simulink model "KD_cl_harness_tomasso"  (R2014b)
settings: Solver=ode45  StartTime=0  StopTime=50  FixedStep=0.01  MaxStep=0.005  RelTol=1e-4  AbsTol=1e-4
InitFcn:
  | load KD_const_coeffs_0624
  | load pexhat_stuff
  | load expcon
  | load thr_ff_map
values from neighbouring files (symbols this model uses):
  c_0 = 0    [expcon.mat]
  c_1 = 1    [expcon.mat]
  c_100 = 100    [expcon.mat]
  c_1000 = 1000    [expcon.mat]
  c_10000 = 10000    [expcon.mat]
  c_1000inv = 0.0010000000475    [expcon.mat]    (also in pexhat_stuff.mat)
  c_100inv = 0.00999999977648    [expcon.mat]
  c_1_int = 1    [expcon.mat]
  c_1d2p4 = 0.416666656733    [expcon.mat]
  c_1p7 = 1.70000004768    [expcon.mat]
  c_4400inv = 0.000227272728807    [pexhat_stuff.mat]
  c_5500inv = 0.000181818177225    [expcon.mat]
  c_80 = 80    [expcon.mat]
  c_90 = 90    [expcon.mat]
  c_cal_phi = 7.6395999713e-06    [expcon.mat]
  c_compmap = [28125.0058594 29577.4082031 31350.1035156 33776.21875 37051.9296875 41026.2695312 45453.9960938 50160.3515625 55029.671875 59986.109375 64980.4296875 69980.4375 ... (320 elements, 20x16)]    [expcon.mat]
  c_ctok = 273.149993896    [expcon.mat]
  c_fflow_max = inf    [expcon.mat]
  c_fflow_min = 0    [expcon.mat]
  c_filt = 0.949999988079    [expcon.mat]
  c_flowdiv = 9.99999974738e-05    [expcon.mat]
  c_flowmin = 0    [expcon.mat]
  c_flowmult = 10000    [expcon.mat]
  c_inf = inf    [expcon.mat]
  c_km1d2k = 0.142857149243    [expcon.mat]
  c_mm3tokgpers = 2.77333338516e-08    [expcon.mat]
  c_n1 = -1    [expcon.mat]
  c_p00001 = 9.99999974738e-06    [expcon.mat]
  c_p01 = 0.00999999977648    [pexhat_stuff.mat]
  c_p016 = 0.01600000076    [expcon.mat]
  c_p1429 = 0.142900004983    [expcon.mat]
  c_p1e9 = 9.99999971718e-10    [expcon.mat]
  c_p4167 = 0.416700005531    [expcon.mat]    (also in pexhat_stuff.mat = 0.416666656733)
  c_p4d1p4 = 0.285714298487    [expcon.mat]
  c_p5401 = 0.540099978447    [expcon.mat]
  c_p9 = 0.899999976158    [expcon.mat]
  c_pincomp = 97.4216003418    [expcon.mat]
  c_ra = 287.002807617    [expcon.mat]
  c_rair = 287.09979248    [expcon.mat]
  c_Rby1000 = 0.000287000002572    [expcon.mat]
  c_roacorr = 8.05689978733e-06    [expcon.mat]
  c_rpmtoradpers = 0.104719758034    [expcon.mat]
  c_svrthrottle1 = [0.924875080585 0.575991511345 0.0858279466629 0.820202827454 0.445821881294 0.509882986546 0.0428557097912 0.753634572029 0]    [expcon.mat]
  c_svrthrottle2 = [0.145454958081 0.14545533061 0.363636374474 0.509091556072 0.509090721607 0.509091317654 0.545454084873 0.618182241917 0.145454272628]    [expcon.mat]
  c_svrthrottlearg = 0.10000000149    [expcon.mat]
  c_svrthrottlebeta = [2282.12670898 -3239.46044922 -142.784469604 -2660.34570312 1434.34350586 4150.43994141 -1580.68164062 -1039.89575195 791.34588623]    [expcon.mat]
  c_ta_max = inf    [expcon.mat]
  c_ta_min = 270    [expcon.mat]
  c_V = 0.0077999997884    [expcon.mat]
  c_vnliftmax = 90    [expcon.mat]
  c_vnliftmin = 40    [expcon.mat]
  Coefs =     [KD_const_coeffs_0624.mat]    (also in pexhat_stuff.mat)
  const =     [KD_const_coeffs_0624.mat]    (also in pexhat_stuff.mat)
  const_exhat =     [pexhat_stuff.mat]
  eegr_map =     [expcon.mat]
  egrr_delay_init = 0    [expcon.mat]
  epim_map =     [expcon.mat]
  eplufin_ff_map =     [expcon.mat]
  expcon =     [expcon.mat]
  invta = [5 5 5 5 2.5 0 0 0 0 0 0 0 ... (240 elements, 16x15)]    [expcon.mat]
  invtacols = [1000 1200 1400 1600 1800 2000 2200 2400 2600 2800 3000 3200 ... (16 elements, 1x16)]    [expcon.mat]
  IV =     [KD_const_coeffs_0624.mat]    (also in pexhat_stuff.mat)
  Lobs_init = [0 0 0]    [expcon.mat]
  map_delay_init = 120    [expcon.mat]
  maxA_t = [51.4567184448 53.8593139648 56.3063011169 58.7576789856 61.1701469421 63.4982337952 65.6955718994 67.7161483765 69.5156555176 71.0527648926 72.2902603149 73.1961746216 ... (16 elements, 1x16)]    [expcon.mat]
  obsA = [0.985195398331  0  0; -0.188821405172  1  0; 0.000342977960827  0  1]    [expcon.mat]
  sample_time = 0.016    [expcon.mat]    (also in pexhat_stuff.mat)
  SVR_EGR =     [KD_const_coeffs_0624.mat]    (also in pexhat_stuff.mat)
  SVR_EGR_exhat =     [pexhat_stuff.mat]
  SVR_throttle =     [KD_const_coeffs_0624.mat]    (also in pexhat_stuff.mat)
  uz_init = [0 0]    [expcon.mat]
undefined symbols (not defined in the file or in its folder): k1_table, k2_table, maxL, minL, Newton, Raphson
libraries: simulink x5
(part 5 of 6)

== system KD_cl_harness_tomasso/ctrl_rb_explicit_20131031_v2/EGR_max_flow/Air_Model_map_use/Forward_Flow ==
  Ro_a : Inport
  Ne_rpm : Inport  Port=2
  Pa : Inport  Port=3
  Pm : Inport  Port=4
  Cal_phi : Subsystem
  Constant2 : Constant  Value=c_p1429  OutDataTypeStr=single
      settings: AttributesFormatString=%<Value>
  Constant3 : Constant  Value=c_1  OutDataTypeStr=single
      settings: AttributesFormatString=%<Value>
  Constant4 : Constant  Value=c_p5401  OutDataTypeStr=single
      settings: AttributesFormatString=%<Value>
  Constant5 : Constant  Value=c_p4167  OutDataTypeStr=single
      settings: AttributesFormatString=%<Value>
  Lookup Table : Lookup  InputValues=invtacols  Table=maxA_t
  Pm_by_Pa : Product  Inputs=*/  SaturateOnIntegerOverflow=on  RndMeth=Zero  InputSameDT=on  OutDataTypeStr=Inherit: Same as first input
  Relational Operator : RelationalOperator  Operator=>  OutDataTypeStr=boolean
      settings: AttributesFormatString=%<Operator>
  Saturation1 : Saturate  UpperLimit=c_1  LowerLimit=c_p4167
      settings: AttributesFormatString=%<UpperLimit>\n%<LowerLimit>
  Saturation2 : Saturate  UpperLimit=c_inf  LowerLimit=c_0
      settings: AttributesFormatString=%<LowerLimit>\n%<UpperLimit>
  Saturation3 : Saturate  UpperLimit=c_inf  LowerLimit=c_100
      settings: AttributesFormatString=%<LowerLimit>\n%<UpperLimit>
  Sqrt : Sqrt  AlgorithmType=Newton-Raphson  SaturateOnIntegerOverflow=on
  Sum : Sum  Inputs=|+-
  Sum1 : Sum  Inputs=|++
  Switch1 : Switch  Criteria=u2 ~= 0
      settings: AttributesFormatString=%<Criteria>
  correct flow1 : Product  Inputs=**  SaturateOnIntegerOverflow=on  RndMeth=Zero  InputSameDT=on  OutDataTypeStr=Inherit: Same as first input
  correct flow2 : Product  Inputs=***  SaturateOnIntegerOverflow=on  RndMeth=Zero  InputSameDT=on  OutDataTypeStr=Inherit: Same as first input
  correct flow3 : Product  Inputs=**  SaturateOnIntegerOverflow=on  RndMeth=Zero  InputSameDT=on  OutDataTypeStr=Inherit: Same as first input
  tokgps1 : Gain  Gain=c_1000inv
  mt_dot_kg_per_s : Outport
  wires:
  Sqrt/1 -> Switch1/1
  correct flow3/1 -> Saturation2/1
  correct flow1/1 -> Sum1/1
  Constant2/1 -> correct flow1/2
  Sum/1 -> correct flow3/1, correct flow1/1
  Constant3/1 -> Sum/1
  Lookup Table/1 -> correct flow2/2  "B_TA"
  Ne_rpm/1 -> Lookup Table/1
  Ro_a/1 -> Cal_phi/2(Ro_a)
  Pa/1 -> [Pa], Saturation3/1
  Pm/1 -> Pm_by_Pa/1
  Pm_by_Pa/1 -> Saturation1/1, Relational Operator/1
  tokgps1/1 -> mt_dot_kg_per_s/1
  correct flow2/1 -> tokgps1/1
  Saturation1/1 -> Sum1/2, Sum/2
  Switch1/1 -> correct flow2/3
  Cal_phi/1(phi) -> correct flow2/1
  Sum1/1 -> correct flow3/2
  [Pa] -> Cal_phi/1(Pa)
  Saturation2/1 -> Sqrt/1
  Saturation3/1 -> Pm_by_Pa/2
  Relational Operator/1 -> Switch1/2
  Constant4/1 -> Switch1/3
  Constant5/1 -> Relational Operator/2

== system KD_cl_harness_tomasso/ctrl_rb_explicit_20131031_v2/While_Iterator_Subsystem/newton/For_Iterator_Subsystem ==
  u : Inport
  sv1 : Inport  Port=2
  sv2 : Inport  Port=3
  arg : Inport  Port=4
  beta : Inport  Port=5
  Demux : Demux  Outputs=2
  Divide : Product  Inputs=*/
  For Iterator : ForIterator  ResetStates=reset  IterationLimit=SVR_EGR_exhat.num_SV
  Gain : Gain  Gain=100
      settings: AttributesFormatString=%<Gain>
  Product{,1..3} (4 alike) : Product  RndMeth=Zero
  Saturation1 : Saturate  UpperLimit=9  LowerLimit=1
      settings: AttributesFormatString=%<LowerLimit>\n%<UpperLimit>
  Selector : Selector  InputPortWidth=SVR_EGR_exhat.num_SV  IndexOptions=Index vector (port)  Indices=[1 3]
  Selector1 : Selector  InputPortWidth=SVR_EGR_exhat.num_SV  IndexOptions=Index vector (port)  Indices=[1 3]
  Selector2 : Selector  InputPortWidth=SVR_EGR_exhat.num_SV  IndexOptions=Index vector (port)  Indices=[1 3]
  Sum : Sum  Inputs=|-+
  Sum1 : Sum  Inputs=+-|
  Sum2 : Sum  Inputs=-|-
  Sum3 : Sum  Inputs=++|
  Unit Delay : UnitDelay  SampleTime=-1
  exp Lookup Table : Lookup  InputValues=SVR_EGR_exhat.exp.x  Table=SVR_EGR_exhat.exp.y  LookUpMeth=Interpolation-Use End Values
      settings: AttributesFormatString=%<LookUpMeth>\n%<InputValues>
  ba : Outport  OutDataTypeStr=single
  wires:
  Saturation1/1 -> [iter]
  For Iterator/1 -> Saturation1/1
  [iter] -> Selector2/2
  [iter] -> Selector1/2
  [iter] -> Selector/2
  Sum3/1 -> ba/1, Unit Delay/1
  Product3/1 -> Sum3/2
  Selector2/1 -> Product3/2
  Gain/1 -> Divide/2
  Product2/1 -> Gain/1
  arg/1 -> Product2/2, Product2/1
  Sum2/1 -> Divide/1
  Product1/1 -> Sum2/2
  Product/1 -> Sum2/1
  Sum1/1 -> Product1/2, Product1/1
  Sum/1 -> Product/2, Product/1
  Demux/2 -> Sum1/1
  Selector1/1 -> Sum1/2
  Demux/1 -> Sum/2
  Selector/1 -> Sum/1
  u/1 -> Demux/1
  beta/1 -> Selector2/1
  sv2/1 -> Selector1/1
  sv1/1 -> Selector/1
  Unit Delay/1 -> Sum3/1
  Divide/1 -> exp Lookup Table/1
  exp Lookup Table/1 -> Product3/1

== system KD_cl_harness_tomasso/ctrl_rb_explicit_20131031_v2/While_Iterator_Subsystem/newton/If_Action_Subsystem ==
  pex : Inport
  ba : Inport  Port=2
  c : Inport  Port=3
  k : Inport  Port=4
  Action Port : ActionPort  ActionType=then
  Gain1 : Gain  Gain=2
  Gain6 : Gain  Gain=2
  Mux : Mux  Inputs=2
  Product : Product  Inputs=***  RndMeth=Zero
  Product1 : Product  Inputs=*/  RndMeth=Zero
  Product2 : Product  Inputs=**  RndMeth=Zero
  Product3 : Product  Inputs=***  RndMeth=Zero
  Product4 : Product  Inputs=*/  RndMeth=Zero
  Saturation1 : Saturate  UpperLimit=inf  LowerLimit=0
      settings: AttributesFormatString=%<LowerLimit>\n%<UpperLimit>
  Saturation2 : Saturate  UpperLimit=inf  LowerLimit=0
      settings: AttributesFormatString=%<LowerLimit>\n%<UpperLimit>
  Saturation3 : Saturate  UpperLimit=c_inf  LowerLimit=c_p1e9
      settings: AttributesFormatString=%<LowerLimit>\n%<UpperLimit>
  Saturation4 : Saturate  UpperLimit=c_inf  LowerLimit=c_p1e9
      settings: AttributesFormatString=%<LowerLimit>\n%<UpperLimit>
  Sqrt1 : Sqrt  AlgorithmType=Newton-Raphson  SaturateOnIntegerOverflow=on
  Sqrt2 : Sqrt  AlgorithmType=Newton-Raphson  SaturateOnIntegerOverflow=on
  Sum1 : Sum  Inputs=++|
  Sum3 : Sum  Inputs=++|
  one : Constant  OutDataTypeStr=single  SampleTime=-1
      settings: AttributesFormatString=%<Value>\n%<SampleTime>
  one1 : Constant  OutDataTypeStr=single  SampleTime=-1
      settings: AttributesFormatString=%<Value>\n%<SampleTime>
  Out : Outport
  wires:
  Saturation4/1 -> Product4/2
  Saturation3/1 -> Product1/2
  Saturation2/1 -> Sqrt1/1
  Saturation1/1 -> Sqrt2/1
  Product3/1 -> Product2/1
  Sqrt1/1 -> Product3/3
  Product4/1 -> Saturation2/1
  Gain1/1 -> Saturation4/1
  Sum1/1 -> Gain1/1
  one1/1 -> Sum1/1
  [k] -> Sum1/2
  [k] -> Product4/1
  [c] -> Product3/2
  [ba] -> Product3/1
  Mux/1 -> Out/1
  Product2/1 -> Mux/2
  Product/1 -> Mux/1
  Sqrt2/1 -> Product/3
  [pex] -> Product2/2
  Product1/1 -> Saturation1/1
  Gain6/1 -> Saturation3/1
  Sum3/1 -> Gain6/1
  one/1 -> Sum3/1
  [k] -> Sum3/2
  [k] -> Product1/1
  [c] -> Product/2
  [ba] -> Product/1
  k/1 -> [k]
  pex/1 -> [pex]
  c/1 -> [c]
  ba/1 -> [ba]

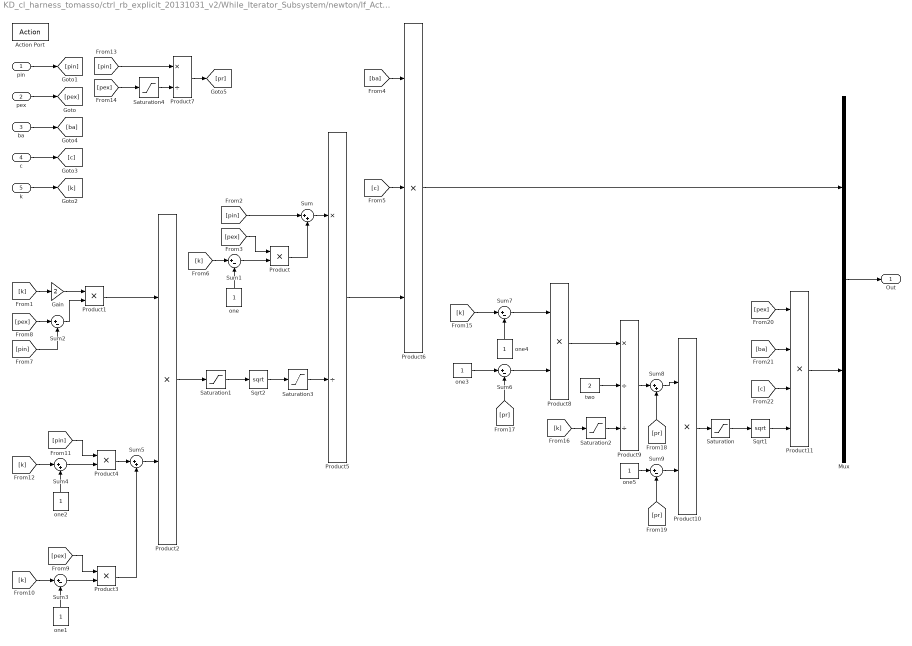
== system KD_cl_harness_tomasso/ctrl_rb_explicit_20131031_v2/While_Iterator_Subsystem/newton/If_Action_Subsystem1 ==
  pin : Inport
  pex : Inport  Port=2
  ba : Inport  Port=3
  c : Inport  Port=4
  k : Inport  Port=5
  Action Port : ActionPort  ActionType=else
  Gain : Gain  Gain=2
  Mux : Mux  Inputs=2
  Product{,1..4} (5 alike) : Product  RndMeth=Zero
  Product10 : Product  Inputs=**  RndMeth=Zero
  Product11 : Product  Inputs=****  RndMeth=Zero
  Product5 : Product  Inputs=*/  RndMeth=Zero
  Product6 : Product  Inputs=***  RndMeth=Zero
  Product7 : Product  Inputs=*/  RndMeth=Zero
  Product8 : Product  Inputs=**  RndMeth=Zero
  Product9 : Product  Inputs=*//  RndMeth=Zero
  Saturation : Saturate  UpperLimit=inf  LowerLimit=0
      settings: AttributesFormatString=%<LowerLimit>\n%<UpperLimit>
  Saturation1 : Saturate  UpperLimit=inf  LowerLimit=0
      settings: AttributesFormatString=%<LowerLimit>\n%<UpperLimit>
  Saturation2 : Saturate  UpperLimit=c_inf  LowerLimit=c_p1e9
      settings: AttributesFormatString=%<LowerLimit>\n%<UpperLimit>
  Saturation3 : Saturate  UpperLimit=c_inf  LowerLimit=c_p00001
      settings: AttributesFormatString=%<LowerLimit>\n%<UpperLimit>
  Saturation4 : Saturate  UpperLimit=c_inf  LowerLimit=c_p1e9
      settings: AttributesFormatString=%<LowerLimit>\n%<UpperLimit>
  Sqrt1 : Sqrt  AlgorithmType=Newton-Raphson  SaturateOnIntegerOverflow=on
  Sqrt2 : Sqrt  AlgorithmType=Newton-Raphson  SaturateOnIntegerOverflow=on
  Sum{,4..5,8} (4 alike) : Sum  Inputs=|++
  Sum{1..3,6..7,9} (6 alike) : Sum  Inputs=|+-
  one{,1..5} (6 alike) : Constant  OutDataTypeStr=single  SampleTime=-1
      settings: AttributesFormatString=%<Value>\n%<SampleTime>
  two : Constant  Value=2  OutDataTypeStr=single  SampleTime=-1
      settings: AttributesFormatString=%<Value>\n%<SampleTime>
  Out : Outport
  wires:
  Saturation4/1 -> Product7/2
  Saturation2/1 -> Product9/3
  Saturation1/1 -> Sqrt2/1
  Saturation/1 -> Sqrt1/1
  Mux/1 -> Out/1
  Product6/1 -> Mux/1
  Product11/1 -> Mux/2
  [c] -> Product11/3
  [ba] -> Product11/2
  [pex] -> Product11/1
  Sqrt1/1 -> Product11/4
  Product10/1 -> Saturation/1
  Sum8/1 -> Product10/1
  [pr] -> Sum9/2
  Sum9/1 -> Product10/2
  one5/1 -> Sum9/1
  [pr] -> Sum8/2
  Product9/1 -> Sum8/1
  [pr] -> Sum6/2
  Product7/1 -> [pr]
  [k] -> Saturation2/1
  two/1 -> Product9/2
  Product8/1 -> Product9/1
  Sum7/1 -> Product8/1
  Sum6/1 -> Product8/2
  one4/1 -> Sum7/2
  [k] -> Sum7/1
  [pex] -> Saturation4/1
  [pin] -> Product7/1
  one3/1 -> Sum6/1
  Product5/1 -> Product6/3
  [c] -> Product6/2
  [ba] -> Product6/1
  Sum/1 -> Product5/1
  Sqrt2/1 -> Saturation3/1
  Product2/1 -> Saturation1/1
  Product3/1 -> Sum5/2
  Product4/1 -> Sum5/1
  Sum5/1 -> Product2/2
  [pin] -> Product4/1
  Sum4/1 -> Product4/2
  [k] -> Sum4/1
  one2/1 -> Sum4/2
  [pex] -> Product3/1
  Sum3/1 -> Product3/2
  [k] -> Sum3/1
  one1/1 -> Sum3/2
  Product1/1 -> Product2/1
  Gain/1 -> Product1/1
  Sum2/1 -> Product1/2
  [pex] -> Sum2/1
  [pin] -> Sum2/2
  [k] -> Gain/1
  Product/1 -> Sum/2
  [pex] -> Product/1
  Sum1/1 -> Product/2
  [k] -> Sum1/1
  one/1 -> Sum1/2
  [pin] -> Sum/1
  pin/1 -> [pin]
  k/1 -> [k]
  c/1 -> [c]
  ba/1 -> [ba]
  pex/1 -> [pex]
  Saturation3/1 -> Product5/2

== system KD_cl_harness_tomasso/ctrl_rb_explicit_20131031_v2/While_Iterator_Subsystem/newton/If_Action_Subsystem2 ==
  pex_hat : Inport
  Action Port : ActionPort  ActionType=else
  pex : Outport
  wires:
  pex_hat/1 -> pex/1

== system KD_cl_harness_tomasso/ctrl_rb_explicit_20131031_v2/While_Iterator_Subsystem/newton/If_Action_Subsystem3 ==
  valve : Inport
  pex_hat : Inport  Port=2
  pex_ecu : Inport  Port=3
  Action Port : ActionPort  ActionType=then
  Divide : Product  Inputs=*/
  Divide1 : Product  Inputs=**
  Divide2 : Product  Inputs=**
  Sum : Sum  Inputs=-+|
  Sum1 : Sum  Inputs=+|+
  fifteen : Constant  Value=15  OutDataTypeStr=single
      settings: AttributesFormatString=%<Value>
  one : Constant  OutDataTypeStr=single
      settings: AttributesFormatString=%<Value>
  pex : Outport
  wires:
  valve/1 -> Divide/1
  fifteen/1 -> Divide/2
  Divide/1 -> Divide1/2, Sum/1
  pex_hat/1 -> Divide1/1
  one/1 -> Sum/2
  Sum/1 -> Divide2/1
  pex_ecu/1 -> Divide2/2
  Divide1/1 -> Sum1/1
  Divide2/1 -> Sum1/2
  Sum1/1 -> pex/1

== system KD_cl_harness_tomasso/ctrl_rb_explicit_20131031_v2/While_Iterator_Subsystem/newton/update ==
  dwdp : Inport
  error : Inport  Port=2
  Data Store Read1 : DataStoreRead  DataStoreName=man_pex_eps
  Data Store Read11 : DataStoreRead  DataStoreName=man_pex_eps
  Data Store Read16 : DataStoreRead  DataStoreName=man_use_LM
  Product2 : Product  Inputs=**  RndMeth=Zero
  Product3 : Product  Inputs=/*  RndMeth=Zero
  Product8 : Product  Inputs=/**  RndMeth=Zero
  Relational Operator7 : RelationalOperator  Operator=>  OutDataTypeStr=boolean
      settings: AttributesFormatString=%<Operator>
  Saturation1 : Saturate  UpperLimit=c_inf  LowerLimit=c_p1e9
      settings: AttributesFormatString=%<LowerLimit>\n%<UpperLimit>
  Saturation3 : Saturate  UpperLimit=c_inf  LowerLimit=c_p1e9
      settings: AttributesFormatString=%<LowerLimit>\n%<UpperLimit>
  Sum1 : Sum  Inputs=|++
  Sum2 : Sum  Inputs=|++
  Switch7 : Switch  Criteria=u2 ~= 0
      settings: AttributesFormatString=%<Criteria>
  man_pex_eps : Gain
  man_pex_eps1 : Gain
  man_use_LM : Gain
  zero8 : Constant  Value=0  OutDataTypeStr=single  SampleTime=-1
      settings: AttributesFormatString=%<Value>\n%<SampleTime>
  delta : Outport
  wires:
  Data Store Read11/1 -> man_pex_eps/1
  Sum2/1 -> Saturation3/1
  Saturation3/1 -> Product8/1
  Product2/1 -> Sum2/2
  error/1 -> [e]
  dwdp/1 -> [dwdp]
  [dwdp] -> Product2/1, Product8/2, Product2/2
  [e] -> Product8/3
  Data Store Read1/1 -> man_pex_eps1/1
  Sum1/1 -> Saturation1/1
  Saturation1/1 -> Product3/1
  [dwdp] -> Sum1/2
  [e] -> Product3/2
  zero8/1 -> Relational Operator7/2
  Data Store Read16/1 -> man_use_LM/1
  Relational Operator7/1 -> Switch7/2
  Product3/1 -> Switch7/3
  Product8/1 -> Switch7/1
  Switch7/1 -> delta/1
  man_pex_eps/1 -> Sum2/1
  man_pex_eps1/1 -> Sum1/1
  man_use_LM/1 -> Relational Operator7/1

== system KD_cl_harness_tomasso/ctrl_rb_explicit_20131031_v2/expcon/find_region/find_region ==
  u : Inport
  IC : Inport  Port=2
  Constant : Constant  DisableCoverage=on  Value=c_0  OutDataTypeStr=Inherit: Inherit via back propagation  PreserveConstantTs=on
      settings: AttributesFormatString=%<Value>
  g_zero_continue : RelationalOperator  Operator=>  OutDataTypeStr=boolean  InputSameDT=on
  get_region_violation : Subsystem
  if_region_1 : SwitchCase
  leq_check : Subsystem
  reg_register : UnitDelay  InitialCondition=c_1_int  SampleTime=-1
      settings: AttributesFormatString=%<X0>
  reg_update_merge : Merge  Inputs=3  InitialOutput=c_1_int
      settings: AttributesFormatString=%<InitialOutput>
  region_1feedthrough : Subsystem  TreatAsAtomicUnit=on
  region_iter : WhileIterator  MaxIters=expcon.Nr  ShowIterationPort=on
  rv_register : UnitDelay  InitialCondition=c_10000  SampleTime=-1
      settings: AttributesFormatString=%<X0>
  rv_update_merge : Merge  Inputs=3  InitialOutput=c_10000
      settings: AttributesFormatString=%<InitialOutput>
  region : Outport  InitialOutput=c_1_int
      settings: AttributesFormatString=%<InitialOutput>
  rv : Outport  Port=2  InitialOutput=c_10000
      settings: AttributesFormatString=%<InitialOutput>
  wires:
  region_iter/1 -> [iter]
  [iter] -> if_region_1/1, get_region_violation/1(region), leq_check/2(region_ind)
  IC/1 -> region_iter/2
  Constant/1 -> g_zero_continue/2
  [reg] -> reg_update_merge/1
  region_1feedthrough/2(region) -> [reg]
  [def] -> leq_check/Action
  if_region_1/2 -> [def]
  [u] -> get_region_violation/2(u)
  u/1 -> [u]
  get_region_violation/1(region_violation) -> region_1feedthrough/1(rvin), leq_check/1(rv_new)
  leq_check/1(rv_update_new) -> rv_update_merge/2
  rv_register/1 -> leq_check/3(rv_old)
  g_zero_continue/1 -> region_iter/1
  leq_check/3(region_update_new) -> reg_update_merge/2
  reg_register/1 -> leq_check/4(region_old)
  reg_update_merge/1 -> reg_register/1, region/1
  rv_update_merge/1 -> g_zero_continue/1, rv_register/1, rv/1
  region_1feedthrough/1(rvout) -> rv_update_merge/1
  if_region_1/1 -> region_1feedthrough/Action
  leq_check/2(rv_update_old) -> rv_update_merge/3
  leq_check/4(region_updateold) -> reg_update_merge/3

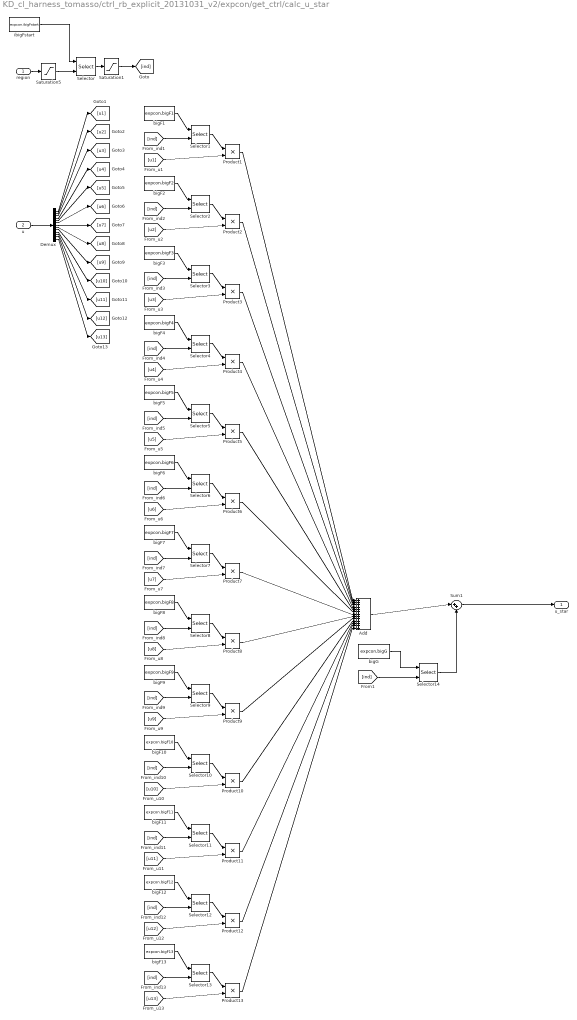
== system KD_cl_harness_tomasso/ctrl_rb_explicit_20131031_v2/expcon/get_ctrl/calc_u_star ==
  region : Inport
  u : Inport  Port=2
  Add : Sum  Inputs=+++++++++++++
  Demux : Demux  Outputs=13
  Product{1..13} (13 alike) : Product  RndMeth=Zero
  Saturation1 : Saturate  UpperLimit=307  LowerLimit=1
      settings: AttributesFormatString=%<LowerLimit>\n%<UpperLimit>
  Saturation5 : Saturate  UpperLimit=103  LowerLimit=1
      settings: AttributesFormatString=%<LowerLimit>\n%<UpperLimit>
  Selector : Selector  InputPortWidth=expcon.Nr  IndexOptions=Index vector (port)  Indices=[1 3]
  Selector{1..14} (14 alike) : Selector  InputPortWidth=309  IndexOptions=Starting index (port)  Indices=[1 3]  OutputSizes=3
  Sum1 : Sum  Inputs=|++
  bigF1 : Constant  Value=expcon.bigF1  OutDataTypeStr=single
      settings: AttributesFormatString=%<Value>
  bigF10 : Constant  Value=expcon.bigF10  OutDataTypeStr=single
      settings: AttributesFormatString=%<Value>
  bigF11 : Constant  Value=expcon.bigF11  OutDataTypeStr=single
      settings: AttributesFormatString=%<Value>
  bigF12 : Constant  Value=expcon.bigF12  OutDataTypeStr=single
      settings: AttributesFormatString=%<Value>
  bigF13 : Constant  Value=expcon.bigF13  OutDataTypeStr=single
      settings: AttributesFormatString=%<Value>
  bigF2 : Constant  Value=expcon.bigF2  OutDataTypeStr=single
      settings: AttributesFormatString=%<Value>
  bigF3 : Constant  Value=expcon.bigF3  OutDataTypeStr=single
      settings: AttributesFormatString=%<Value>
  bigF4 : Constant  Value=expcon.bigF4  OutDataTypeStr=single
      settings: AttributesFormatString=%<Value>
  bigF5 : Constant  Value=expcon.bigF5  OutDataTypeStr=single
      settings: AttributesFormatString=%<Value>
  bigF6 : Constant  Value=expcon.bigF6  OutDataTypeStr=single
      settings: AttributesFormatString=%<Value>
  bigF7 : Constant  Value=expcon.bigF7  OutDataTypeStr=single
      settings: AttributesFormatString=%<Value>
  bigF8 : Constant  Value=expcon.bigF8  OutDataTypeStr=single
      settings: AttributesFormatString=%<Value>
  bigF9 : Constant  Value=expcon.bigF9  OutDataTypeStr=single
      settings: AttributesFormatString=%<Value>
  bigG : Constant  Value=expcon.bigG  OutDataTypeStr=single
      settings: AttributesFormatString=%<Value>
  ibigFstart : Constant  Value=expcon.ibigFstart  OutDataTypeStr=single
      settings: AttributesFormatString=%<Value>
  u_star : Outport
  wires:
  Product13/1 -> Add/13
  [u13] -> Product13/2
  Selector13/1 -> Product13/1
  [ind] -> Selector13/2
  bigF13/1 -> Selector13/1
  Demux/13 -> [u13]
  Product12/1 -> Add/12
  [u12] -> Product12/2
  Selector12/1 -> Product12/1
  [ind] -> Selector12/2
  bigF12/1 -> Selector12/1
  Demux/12 -> [u12]
  Product11/1 -> Add/11
  [u11] -> Product11/2
  Selector11/1 -> Product11/1
  [ind] -> Selector11/2
  bigF11/1 -> Selector11/1
  Demux/11 -> [u11]
  Product10/1 -> Add/10
  [u10] -> Product10/2
  Selector10/1 -> Product10/1
  [ind] -> Selector10/2
  bigF10/1 -> Selector10/1
  Demux/10 -> [u10]
  Product9/1 -> Add/9
  [u9] -> Product9/2
  Selector9/1 -> Product9/1
  [ind] -> Selector9/2
  bigF9/1 -> Selector9/1
  Demux/9 -> [u9]
  Product8/1 -> Add/8
  [u8] -> Product8/2
  Selector8/1 -> Product8/1
  [ind] -> Selector8/2
  bigF8/1 -> Selector8/1
  Demux/8 -> [u8]
  Product7/1 -> Add/7
  [u7] -> Product7/2
  Selector7/1 -> Product7/1
  [ind] -> Selector7/2
  bigF7/1 -> Selector7/1
  Demux/7 -> [u7]
  Product6/1 -> Add/6
  [u6] -> Product6/2
  Selector6/1 -> Product6/1
  [ind] -> Selector6/2
  bigF6/1 -> Selector6/1
  Demux/6 -> [u6]
  Product5/1 -> Add/5
  [u5] -> Product5/2
  Selector5/1 -> Product5/1
  [ind] -> Selector5/2
  bigF5/1 -> Selector5/1
  Demux/5 -> [u5]
  Product4/1 -> Add/4
  [u4] -> Product4/2
  Selector4/1 -> Product4/1
  [ind] -> Selector4/2
  bigF4/1 -> Selector4/1
  Demux/4 -> [u4]
  Product3/1 -> Add/3
  [u3] -> Product3/2
  Selector3/1 -> Product3/1
  [ind] -> Selector3/2
  bigF3/1 -> Selector3/1
  Demux/3 -> [u3]
  Product2/1 -> Add/2
  [u2] -> Product2/2
  Selector2/1 -> Product2/1
  [ind] -> Selector2/2
  bigF2/1 -> Selector2/1
  Demux/2 -> [u2]
  Product1/1 -> Add/1
  [u1] -> Product1/2
  Selector1/1 -> Product1/1
  [ind] -> Selector1/2
  bigF1/1 -> Selector1/1
  Demux/1 -> [u1]
  Saturation1/1 -> [ind]
  Saturation5/1 -> Selector/2
  Add/1 -> Sum1/1
  [ind] -> Selector14/2
  u/1 -> Demux/1
  Selector14/1 -> Sum1/2
  bigG/1 -> Selector14/1
  Sum1/1 -> u_star/1
  Selector/1 -> Saturation1/1
  ibigFstart/1 -> Selector/1
  region/1 -> Saturation5/1

== system KD_cl_harness_tomasso/ctrl_rb_explicit_20131031_v2/invert_flow/valve_inversion/Cal_phi1 ==
  Pa : Inport
  Ro_a : Inport  Port=2
  Abs : Abs
  Gain1 : Gain  Gain=c_cal_phi  SaturateOnIntegerOverflow=on  OutDataTypeStr=Inherit: Same as input  ParamDataTypeStr=Inherit: Same as input
  Product4 : Product  Inputs=**  SaturateOnIntegerOverflow=on  RndMeth=Zero  InputSameDT=on  OutDataTypeStr=Inherit: Same as first input
  Sqrt : Sqrt  AlgorithmType=Newton-Raphson  SaturateOnIntegerOverflow=on
  phi : Outport
  wires:
  Abs/1 -> Sqrt/1
  Gain1/1 -> Abs/1
  Sqrt/1 -> phi/1
  Ro_a/1 -> Product4/2
  Pa/1 -> Product4/1
  Product4/1 -> Gain1/1

== system KD_cl_harness_tomasso/ctrl_rb_explicit_20131031_v2/ntestimator/Throttle_Model/Air_Model_map_use ==
  TA_deg : Inport
  Ne_rpm : Inport  Port=2
  Pim_Pa : Inport  Port=3
  Ta_K : Inport  Port=4
  R_a : Inport  Port=5
  wegrthr : Inport  Port=6
  Forward_Flow : Subsystem
  Product1 : Product  Inputs=*//  SaturateOnIntegerOverflow=on  RndMeth=Zero  InputSameDT=on  OutDataTypeStr=Inherit: Same as first input
  Saturation1 : Saturate  UpperLimit=c_inf  LowerLimit=c_p1e9
      settings: AttributesFormatString=%<LowerLimit>\n%<UpperLimit>
  Saturation5 : Saturate  UpperLimit=c_inf  LowerLimit=c_p1e9
      settings: AttributesFormatString=%<LowerLimit>\n%<UpperLimit>
  one : Constant  OutDataTypeStr=single  SampleTime=sample_time
      settings: AttributesFormatString=%<Value>\n%<SampleTime>
  p_pre_throttle : Outport
  wires:
  Product1/1 -> Forward_Flow/1(Ro_a)
  TA_deg/1 -> Forward_Flow/2(TA_deg)
  Pim_Pa/1 -> Forward_Flow/4(Pm)
  Ta_K/1 -> Saturation5/1
  R_a/1 -> Saturation1/1
  one/1 -> Product1/1
  Ne_rpm/1 -> Forward_Flow/3(Ne_rpm)
  wegrthr/1 -> Forward_Flow/5(wegrthr)
  Forward_Flow/1(p_pre_throttle) -> p_pre_throttle/1
  Saturation5/1 -> Product1/2
  Saturation1/1 -> Product1/3

== system KD_cl_harness_tomasso/ctrl_rb_explicit_20131031_v2/set_point_maps/intake_pressure_map/boost_pressure_map ==
  fuel_rate_mm3perst : Inport
  engine_speed : Inport  Port=2
  epimbs_map : Lookup2D  RowIndex=epim_map.x  ColumnIndex=epim_map.y  Table=epim_map.z  LookUpMeth=Interpolation-Use End Values
      settings: AttributesFormatString=%<LookUpMeth>\n%<RowIndex>\n%<ColumnIndex>
  intake_manifold_pressure : Outport
  wires:
  epimbs_map/1 -> intake_manifold_pressure/1
  fuel_rate_mm3perst/1 -> epimbs_map/2
  engine_speed/1 -> epimbs_map/1

== system KD_cl_harness_tomasso/EGR Throttle/EGR Throttle/Throttle Model2/Air Model_map_use/Back-Flow ==
  TA[deg] : Inport
  Ne[rpm] : Inport  Port=2
  Ro_m : Inport  Port=3
  Pa : Inport  Port=4
  Pm : Inport  Port=5
  Cal phi1 : Subsystem
  Constant1 : Constant  Value=(const.k/(2*(const.k+1)))^0.5
  Constant2 : Constant  Value=SVR_throttle.Beta
  Constant6 : Constant  Value=SVR_throttle.num_SV
  Constant7 : Constant  Value=SVR_throttle.SV
  Constant8 : Constant  Value=SVR_throttle.arg
  Gain : Gain  Gain=1/100
  Gain1 : Gain  Gain=1/5500
  Mux : Mux  Inputs=2
  Phi1 : Fcn  Expr=sqrt(((const.k-1)/(2*const.k)*(1-u)+u)*(1-u))
  Pm/Pa1 : Product  Inputs=/*  SaturateOnIntegerOverflow=on  RndMeth=Zero  InputSameDT=on  OutDataTypeStr=Inherit: Same as first input
  SVR_throttle : MATLAB Function  TreatAsAtomicUnit=on
  Saturation : Saturate  UpperLimit=inf  LowerLimit=0
  Saturation1 : Saturate  UpperLimit=1.0  LowerLimit=1/(const.k+1)
  Switch1 : Switch  Criteria=u2 > Threshold  Threshold=1/(const.k+1)
  correct flow2 : Product  Inputs=***  SaturateOnIntegerOverflow=on  RndMeth=Zero  InputSameDT=on  OutDataTypeStr=Inherit: Same as first input
  tokgps1 : Gain  Gain=1/1000
  mt_dot[kg/s] : Outport
  wires:
  Cal phi1/1(phi) -> correct flow2/1
  Constant1/1 -> Switch1/3
  Switch1/1 -> correct flow2/3
  Saturation1/1 -> Phi1/1
  Phi1/1 -> Switch1/1
  correct flow2/1 -> tokgps1/1
  tokgps1/1 -> mt_dot[kg/s]/1
  Pm/Pa1/1 -> Switch1/2, Saturation1/1
  Pm/1 -> Pm/Pa1/1, Cal phi1/1(Pm)
  Pa/1 -> Pm/Pa1/2
  Ro_m/1 -> Cal phi1/2(Ro_m)
  SVR_throttle/1(B_A_spd) -> Saturation/1
  TA[deg]/1 -> Gain/1
  Gain/1 -> Mux/1
  Gain1/1 -> Mux/2
  Ne[rpm]/1 -> Gain1/1
  Constant6/1 -> SVR_throttle/2(num_SV)
  Constant2/1 -> SVR_throttle/3(Beta)
  Constant7/1 -> SVR_throttle/4(SV)
  Constant8/1 -> SVR_throttle/5(arg)
  Mux/1 -> SVR_throttle/1(u)
  Saturation/1 -> correct flow2/2

== system KD_cl_harness_tomasso/EGR Throttle/EGR Throttle/Throttle Model2/Air Model_map_use/Forward-Flow ==
  Ro_a : Inport
  TA[deg] : Inport  Port=2
  Ne[rpm] : Inport  Port=3
  Pa : Inport  Port=4
  Pm : Inport  Port=5
  Cal phi : Subsystem
  Constant1 : Constant  Value=(const.k/(2*(const.k+1)))^0.5
  Constant2 : Constant  Value=SVR_throttle.Beta
  Constant6 : Constant  Value=SVR_throttle.num_SV
  Constant7 : Constant  Value=SVR_throttle.SV
  Constant8 : Constant  Value=SVR_throttle.arg
  Gain : Gain  Gain=1/100
  Gain1 : Gain  Gain=1/5500
  Mux : Mux  Inputs=2
  Phi1 : Fcn  Expr=sqrt(((const.k-1)/(2*const.k)*(1-u)+u)*(1-u))
  Pm/Pa1 : Product  Inputs=*/  SaturateOnIntegerOverflow=on  RndMeth=Zero  InputSameDT=on  OutDataTypeStr=Inherit: Same as first input
  SVR_throttle : MATLAB Function  TreatAsAtomicUnit=on
  Saturation : Saturate  UpperLimit=inf  LowerLimit=0
  Saturation1 : Saturate  UpperLimit=1.0  LowerLimit=1/(const.k+1)
  Switch1 : Switch  Criteria=u2 > Threshold  Threshold=1/(const.k+1)
  correct flow2 : Product  Inputs=***  SaturateOnIntegerOverflow=on  RndMeth=Zero  InputSameDT=on  OutDataTypeStr=Inherit: Same as first input
  tokgps1 : Gain  Gain=1/1000
  mt_dot[kg/s] : Outport
  wires:
  Cal phi/1(phi) -> correct flow2/1
  Constant1/1 -> Switch1/3
  Switch1/1 -> correct flow2/3
  Saturation1/1 -> Phi1/1
  Phi1/1 -> Switch1/1
  correct flow2/1 -> tokgps1/1
  tokgps1/1 -> mt_dot[kg/s]/1
  Pm/Pa1/1 -> Switch1/2, Saturation1/1
  Pm/1 -> Pm/Pa1/1
  Pa/1 -> Pm/Pa1/2, Cal phi/1(Pa)
  Ro_a/1 -> Cal phi/2(Ro_a)
  Mux/1 -> SVR_throttle/1(u)
  TA[deg]/1 -> Gain/1
  Gain/1 -> Mux/1
  Gain1/1 -> Mux/2
  Ne[rpm]/1 -> Gain1/1
  SVR_throttle/1(B_A_spd) -> Saturation/1
  Constant6/1 -> SVR_throttle/2(num_SV)
  Constant2/1 -> SVR_throttle/3(Beta)
  Constant7/1 -> SVR_throttle/4(SV)
  Constant8/1 -> SVR_throttle/5(arg)
  Saturation/1 -> correct flow2/2  "B(TA)(g/s)"

== system KD_cl_harness_tomasso/EGR Valve/SVR EGR/EGR_model/Air Model_map_use/Back-Flow ==
  TA[deg] : Inport
  Ne[rpm] : Inport  Port=2
  Ro_m : Inport  Port=3
  Pa : Inport  Port=4
  Pm : Inport  Port=5
  Cal phi1 : Subsystem
  Constant1 : Constant  Value=(const.k/(2*(const.k+1)))^0.5
  Constant2 : Constant  Value=SVR_EGR.Beta
  Constant6 : Constant  Value=SVR_EGR.num_SV
  Constant7 : Constant  Value=SVR_EGR.SV
  Constant8 : Constant  Value=SVR_EGR.arg
  Gain : Gain  Gain=1/100
  Gain1 : Gain  Gain=1/5500
  Gain2 : Gain  Gain=1/1000
  Mux : Mux  Inputs=2
  Phi1 : Fcn  Expr=sqrt(((const.k-1)/(2*const.k)*(1-u)+u)*(1-u))
  Pm/Pa1 : Product  Inputs=/*  SaturateOnIntegerOverflow=on  RndMeth=Zero  InputSameDT=on  OutDataTypeStr=Inherit: Same as first input
  SVR_EGR : MATLAB Function  TreatAsAtomicUnit=on
  Saturation : Saturate  UpperLimit=inf  LowerLimit=0
  Saturation1 : Saturate  UpperLimit=1.0  LowerLimit=1/(const.k+1)
  Switch1 : Switch  Criteria=u2 > Threshold  Threshold=1/(const.k+1)
  correct flow2 : Product  Inputs=***  SaturateOnIntegerOverflow=on  RndMeth=Zero  InputSameDT=on  OutDataTypeStr=Inherit: Same as first input
  mt_dot[kg/s] : Outport
  wires:
  Gain2/1 -> mt_dot[kg/s]/1
  Mux/1 -> SVR_EGR/1(u)
  Constant8/1 -> SVR_EGR/5(arg)
  Constant7/1 -> SVR_EGR/4(SV)
  Constant2/1 -> SVR_EGR/3(Beta)
  Constant6/1 -> SVR_EGR/2(num_SV)
  Ne[rpm]/1 -> Gain1/1
  Gain1/1 -> Mux/2
  Gain/1 -> Mux/1
  TA[deg]/1 -> Gain/1
  SVR_EGR/1(B_A_spd) -> Saturation/1
  Ro_m/1 -> Cal phi1/2(Ro_m)
  Pa/1 -> Pm/Pa1/2
  Pm/1 -> Cal phi1/1(Pm), Pm/Pa1/1
  Pm/Pa1/1 -> Saturation1/1, Switch1/2
  correct flow2/1 -> Gain2/1
  Phi1/1 -> Switch1/1
  Saturation1/1 -> Phi1/1
  Switch1/1 -> correct flow2/3
  Constant1/1 -> Switch1/3
  Cal phi1/1(phi) -> correct flow2/1
  Saturation/1 -> correct flow2/2

== system KD_cl_harness_tomasso/EGR Valve/SVR EGR/EGR_model/Air Model_map_use/Forward-Flow ==
  Ro_a : Inport
  TA[deg] : Inport  Port=2
  Ne[rpm] : Inport  Port=3
  Pa : Inport  Port=4
  Pm : Inport  Port=5
  Cal phi : Subsystem
  Constant1 : Constant  Value=(const.k/(2*(const.k+1)))^0.5
  Constant3 : Constant  Value=SVR_EGR.Beta
  Constant4 : Constant  Value=SVR_EGR.num_SV
  Constant5 : Constant  Value=SVR_EGR.SV
  Constant9 : Constant  Value=SVR_EGR.arg
  Gain : Gain  Gain=1/100
  Gain1 : Gain  Gain=1/4400
  Gain2 : Gain  Gain=1/1000
  Mux : Mux  Inputs=2
  Phi1 : Fcn  Expr=sqrt(((const.k-1)/(2*const.k)*(1-u)+u)*(1-u))
  Pm/Pa1 : Product  Inputs=*/  SaturateOnIntegerOverflow=on  RndMeth=Zero  InputSameDT=on  OutDataTypeStr=Inherit: Same as first input
  SVR_EGR : MATLAB Function  TreatAsAtomicUnit=on
  Saturation : Saturate  UpperLimit=inf  LowerLimit=0
  Saturation1 : Saturate  UpperLimit=1.0  LowerLimit=1/(const.k+1)
  Switch1 : Switch  Criteria=u2 > Threshold  Threshold=1/(const.k+1)
  correct flow2 : Product  Inputs=***  SaturateOnIntegerOverflow=on  RndMeth=Zero  InputSameDT=on  OutDataTypeStr=Inherit: Same as first input
  mt_dot[kg/s] : Outport
  wires:
  Gain2/1 -> mt_dot[kg/s]/1
  Constant9/1 -> SVR_EGR/5(arg)
  Constant5/1 -> SVR_EGR/4(SV)
  Constant3/1 -> SVR_EGR/3(Beta)
  Constant4/1 -> SVR_EGR/2(num_SV)
  SVR_EGR/1(B_A_spd) -> Saturation/1
  Ne[rpm]/1 -> Gain1/1
  Gain1/1 -> Mux/2
  Gain/1 -> Mux/1
  TA[deg]/1 -> Gain/1
  Mux/1 -> SVR_EGR/1(u)
  Ro_a/1 -> Cal phi/2(Ro_a)
  Pa/1 -> Cal phi/1(Pa), Pm/Pa1/2
  Pm/1 -> Pm/Pa1/1
  Pm/Pa1/1 -> Saturation1/1, Switch1/2
  correct flow2/1 -> Gain2/1
  Phi1/1 -> Switch1/1
  Saturation1/1 -> Phi1/1
  Switch1/1 -> correct flow2/3
  Constant1/1 -> Switch1/3
  Cal phi/1(phi) -> correct flow2/1
  Saturation/1 -> correct flow2/2  "B(TA)(g/s)"

== system KD_cl_harness_tomasso/ctrl_rb_explicit_20131031_v2/EGR_max_flow/Air_Model_map_use/Forward_Flow/Cal_phi ==
  Pa : Inport
  Ro_a : Inport  Port=2
  Abs : Abs
  Gain2 : Gain  Gain=c_cal_phi  ParamDataTypeStr=single  SaturateOnIntegerOverflow=on  OutDataTypeStr=Inherit: Same as input
  Product4 : Product  Inputs=**  OutDataTypeStr=single  SaturateOnIntegerOverflow=on  RndMeth=Zero  InputSameDT=on
  Sqrt : Sqrt  AlgorithmType=Newton-Raphson  SaturateOnIntegerOverflow=on
  phi : Outport
  wires:
  Sqrt/1 -> phi/1
  Abs/1 -> Sqrt/1
  Product4/1 -> Gain2/1
  Gain2/1 -> Abs/1
  Pa/1 -> Product4/1
  Ro_a/1 -> Product4/2

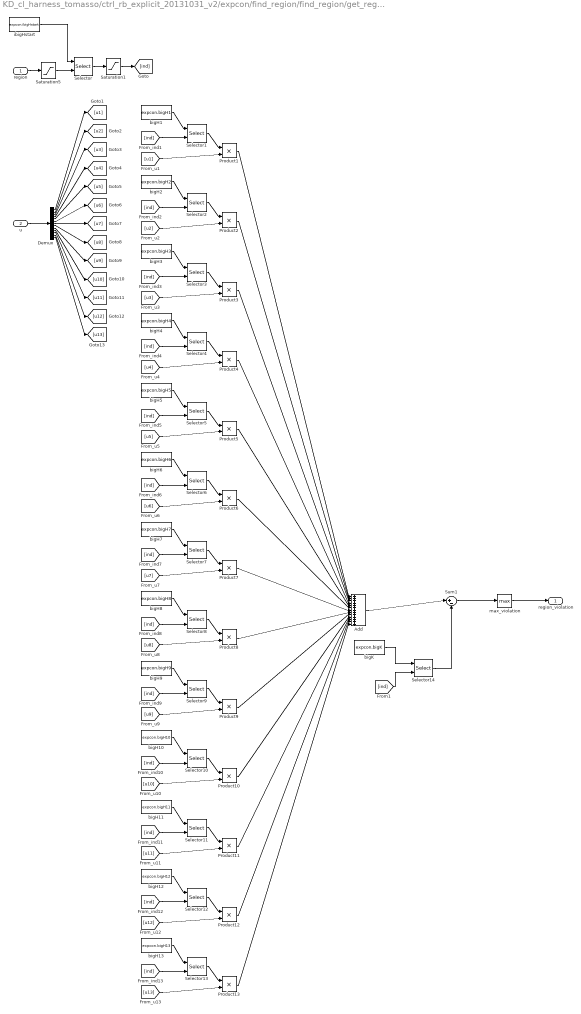
== system KD_cl_harness_tomasso/ctrl_rb_explicit_20131031_v2/expcon/find_region/find_region/get_region_violation ==
  region : Inport
  u : Inport  Port=2
  Add : Sum  Inputs=+++++++++++++
  Demux : Demux  Outputs=13
  Product{1..13} (13 alike) : Product  RndMeth=Zero
  Saturation1 : Saturate  UpperLimit=1021  LowerLimit=1
      settings: AttributesFormatString=%<LowerLimit>\n%<UpperLimit>
  Saturation5 : Saturate  UpperLimit=103  LowerLimit=1
      settings: AttributesFormatString=%<LowerLimit>\n%<UpperLimit>
  Selector : Selector  InputPortWidth=expcon.Nr  IndexOptions=Index vector (port)  Indices=[1 3]
  Selector{1..14} (14 alike) : Selector  InputPortWidth=1030  IndexOptions=Starting index (port)  Indices=[1 3]  OutputSizes=10
  Sum1 : Sum  Inputs=|+-
  bigH1 : Constant  Value=expcon.bigH1  OutDataTypeStr=single
      settings: AttributesFormatString=%<Value>
  bigH10 : Constant  Value=expcon.bigH10  OutDataTypeStr=single
      settings: AttributesFormatString=%<Value>
  bigH11 : Constant  Value=expcon.bigH11  OutDataTypeStr=single
      settings: AttributesFormatString=%<Value>
  bigH12 : Constant  Value=expcon.bigH12  OutDataTypeStr=single
      settings: AttributesFormatString=%<Value>
  bigH13 : Constant  Value=expcon.bigH13  OutDataTypeStr=single
      settings: AttributesFormatString=%<Value>
  bigH2 : Constant  Value=expcon.bigH2  OutDataTypeStr=single
      settings: AttributesFormatString=%<Value>
  bigH3 : Constant  Value=expcon.bigH3  OutDataTypeStr=single
      settings: AttributesFormatString=%<Value>
  bigH4 : Constant  Value=expcon.bigH4  OutDataTypeStr=single
      settings: AttributesFormatString=%<Value>
  bigH5 : Constant  Value=expcon.bigH5  OutDataTypeStr=single
      settings: AttributesFormatString=%<Value>
  bigH6 : Constant  Value=expcon.bigH6  OutDataTypeStr=single
      settings: AttributesFormatString=%<Value>
  bigH7 : Constant  Value=expcon.bigH7  OutDataTypeStr=single
      settings: AttributesFormatString=%<Value>
  bigH8 : Constant  Value=expcon.bigH8  OutDataTypeStr=single
      settings: AttributesFormatString=%<Value>
  bigH9 : Constant  Value=expcon.bigH9  OutDataTypeStr=single
      settings: AttributesFormatString=%<Value>
  bigK : Constant  Value=expcon.bigK  OutDataTypeStr=single
      settings: AttributesFormatString=%<Value>
  ibigHstart : Constant  Value=expcon.ibigHstart  OutDataTypeStr=single
      settings: AttributesFormatString=%<Value>
  max_violation : MinMax  Function=max
      settings: AttributesFormatString=%<Function>
  region_violation : Outport
  wires:
  Product13/1 -> Add/13
  [u13] -> Product13/2
  Selector13/1 -> Product13/1
  [ind] -> Selector13/2
  bigH13/1 -> Selector13/1
  Demux/13 -> [u13]
  Product12/1 -> Add/12
  [u12] -> Product12/2
  Selector12/1 -> Product12/1
  [ind] -> Selector12/2
  bigH12/1 -> Selector12/1
  Demux/12 -> [u12]
  Product11/1 -> Add/11
  [u11] -> Product11/2
  Selector11/1 -> Product11/1
  [ind] -> Selector11/2
  bigH11/1 -> Selector11/1
  Demux/11 -> [u11]
  Product10/1 -> Add/10
  [u10] -> Product10/2
  Selector10/1 -> Product10/1
  [ind] -> Selector10/2
  bigH10/1 -> Selector10/1
  Demux/10 -> [u10]
  Product9/1 -> Add/9
  [u9] -> Product9/2
  Selector9/1 -> Product9/1
  [ind] -> Selector9/2
  bigH9/1 -> Selector9/1
  Demux/9 -> [u9]
  Product8/1 -> Add/8
  [u8] -> Product8/2
  Selector8/1 -> Product8/1
  [ind] -> Selector8/2
  bigH8/1 -> Selector8/1
  Demux/8 -> [u8]
  Product7/1 -> Add/7
  [u7] -> Product7/2
  Selector7/1 -> Product7/1
  [ind] -> Selector7/2
  bigH7/1 -> Selector7/1
  Demux/7 -> [u7]
  Product6/1 -> Add/6
  [u6] -> Product6/2
  Selector6/1 -> Product6/1
  [ind] -> Selector6/2
  bigH6/1 -> Selector6/1
  Demux/6 -> [u6]
  Product5/1 -> Add/5
  [u5] -> Product5/2
  Selector5/1 -> Product5/1
  [ind] -> Selector5/2
  bigH5/1 -> Selector5/1
  Demux/5 -> [u5]
  Product4/1 -> Add/4
  [u4] -> Product4/2
  Selector4/1 -> Product4/1
  [ind] -> Selector4/2
  bigH4/1 -> Selector4/1
  Demux/4 -> [u4]
  Product3/1 -> Add/3
  [u3] -> Product3/2
  Selector3/1 -> Product3/1
  [ind] -> Selector3/2
  bigH3/1 -> Selector3/1
  Demux/3 -> [u3]
  Product2/1 -> Add/2
  [u2] -> Product2/2
  Selector2/1 -> Product2/1
  [ind] -> Selector2/2
  bigH2/1 -> Selector2/1
  Demux/2 -> [u2]
  Product1/1 -> Add/1
  [u1] -> Product1/2
  Selector1/1 -> Product1/1
  [ind] -> Selector1/2
  bigH1/1 -> Selector1/1
  Demux/1 -> [u1]
  Saturation1/1 -> [ind]
  Saturation5/1 -> Selector/2
  Add/1 -> Sum1/1
  [ind] -> Selector14/2
  u/1 -> Demux/1
  Selector14/1 -> Sum1/2
  bigK/1 -> Selector14/1
  max_violation/1 -> region_violation/1
  Sum1/1 -> max_violation/1
  Selector/1 -> Saturation1/1
  ibigHstart/1 -> Selector/1
  region/1 -> Saturation5/1

== system KD_cl_harness_tomasso/ctrl_rb_explicit_20131031_v2/expcon/find_region/find_region/leq_check ==
  rv_new : Inport
  region_ind : Inport  Port=2
  rv_old : Inport  Port=3
  region_old : Inport  Port=4
  Action Port : ActionPort  ActionType=default
  if_new_min_rv : If  NumInputs=2  IfExpression=u1 < u2
  new_region : Subsystem  TreatAsAtomicUnit=on
  old_region : Subsystem  TreatAsAtomicUnit=on
  rv_update_new : Outport
  rv_update_old : Outport  Port=2
  region_update_new : Outport  Port=3
  region_updateold : Outport  Port=4
  wires:
  if_new_min_rv/2 -> [els]
  [els] -> old_region/Action
  [rv] -> if_new_min_rv/2
  rv_old/1 -> old_region/1(rv_in), [rv]
  rv_new/1 -> if_new_min_rv/1, new_region/1(rv_in)
  if_new_min_rv/1 -> new_region/Action
  region_ind/1 -> new_region/2(region_in)
  new_region/1(rv_out) -> rv_update_new/1
  region_old/1 -> old_region/2(region_in)
  new_region/2(region_out) -> region_update_new/1
  old_region/1(rv_out) -> rv_update_old/1
  old_region/2(region_out) -> region_updateold/1

== system KD_cl_harness_tomasso/ctrl_rb_explicit_20131031_v2/expcon/find_region/find_region/region_1feedthrough ==
  rvin : Inport
  Action Port : ActionPort  ActionType=case
  region_1 : Constant  Value=c_1_int  OutDataTypeStr=int32
  rvout : Outport
  region : Outport  Port=2  InitialOutput=1
      settings: AttributesFormatString=%<InitialOutput>
  wires:
  rvin/1 -> rvout/1
  region_1/1 -> region/1

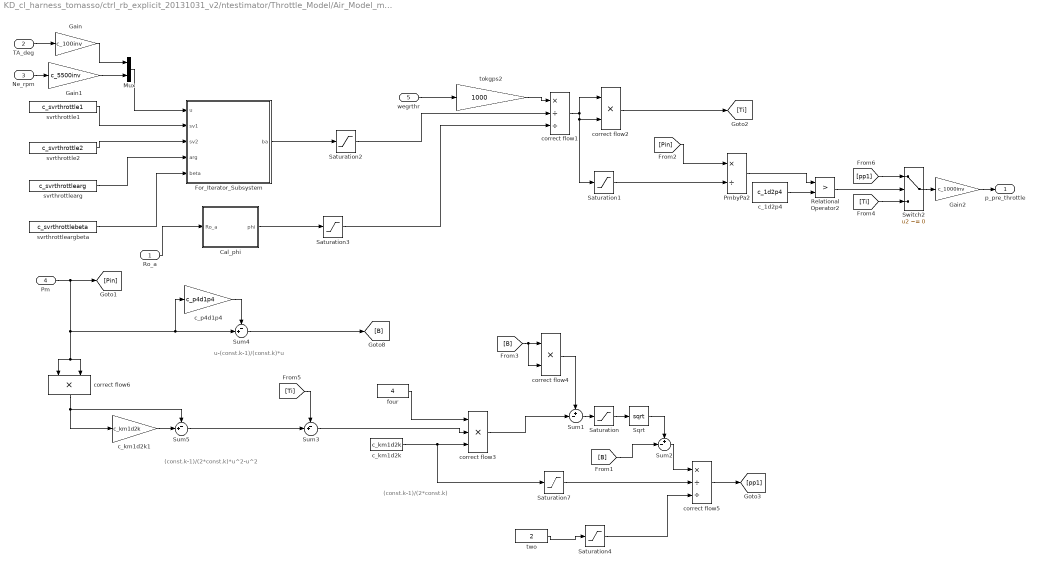
== system KD_cl_harness_tomasso/ctrl_rb_explicit_20131031_v2/ntestimator/Throttle_Model/Air_Model_map_use/Forward_Flow ==
  note: u-(const.k-1)/(const.k)*u
  note: (const.k-1)/(2*const.k)*u^2-u^2
  note: (const.k-1)/(2*const.k)
  Ro_a : Inport
  TA_deg : Inport  Port=2
  Ne_rpm : Inport  Port=3
  Pm : Inport  Port=4
  wegrthr : Inport  Port=5
  Cal_phi : Subsystem
  For_Iterator_Subsystem : Subsystem  TreatAsAtomicUnit=on
  Gain : Gain  Gain=c_100inv
      settings: AttributesFormatString=%<Gain>
  Gain1 : Gain  Gain=c_5500inv
      settings: AttributesFormatString=%<Gain>
  Gain2 : Gain  Gain=c_1000inv
      settings: AttributesFormatString=%<Gain>
  Mux : Mux  Inputs=2
  PmbyPa2 : Product  Inputs=*/  SaturateOnIntegerOverflow=on  RndMeth=Zero  InputSameDT=on  OutDataTypeStr=Inherit: Same as first input
  Relational Operator2 : RelationalOperator  Operator=>  OutDataTypeStr=boolean
      settings: AttributesFormatString=%<Operator>
  Saturation : Saturate  UpperLimit=c_inf  LowerLimit=0
      settings: AttributesFormatString=%<LowerLimit>\n%<UpperLimit>
  Saturation{1..4,7} (5 alike) : Saturate  UpperLimit=c_inf  LowerLimit=c_p1e9
      settings: AttributesFormatString=%<LowerLimit>\n%<UpperLimit>
  Sqrt : Sqrt  AlgorithmType=Newton-Raphson  SaturateOnIntegerOverflow=on
  Sum1 : Sum  Inputs=+-|
  Sum2 : Sum  Inputs=+-|
  Sum3 : Sum  Inputs=-+|
  Sum4 : Sum  Inputs=-+|
  Sum5 : Sum  Inputs=-+|
  Switch2 : Switch  Criteria=u2 ~= 0
      settings: AttributesFormatString=%<Criteria>
  c_1d2p4 : Constant  Value=c_1d2p4  OutDataTypeStr=single  SampleTime=sample_time
      settings: AttributesFormatString=%<Value>\n%<SampleTime>
  c_km1d2k : Constant  Value=c_km1d2k  OutDataTypeStr=single  SampleTime=sample_time
      settings: AttributesFormatString=%<Value>\n%<SampleTime>
  c_km1d2k1 : Gain  Gain=c_km1d2k
  c_p4d1p4 : Gain  Gain=c_p4d1p4
  correct flow1 : Product  Inputs=*//  SaturateOnIntegerOverflow=on  RndMeth=Zero  InputSameDT=on  OutDataTypeStr=Inherit: Same as first input
  correct flow2 : Product  Inputs=**  SaturateOnIntegerOverflow=on  RndMeth=Zero  InputSameDT=on  OutDataTypeStr=Inherit: Same as first input
  correct flow3 : Product  Inputs=***  SaturateOnIntegerOverflow=on  RndMeth=Zero  InputSameDT=on  OutDataTypeStr=Inherit: Same as first input
  correct flow4 : Product  Inputs=**  SaturateOnIntegerOverflow=on  RndMeth=Zero  InputSameDT=on  OutDataTypeStr=Inherit: Same as first input
  correct flow5 : Product  Inputs=*//  SaturateOnIntegerOverflow=on  RndMeth=Zero  InputSameDT=on  OutDataTypeStr=Inherit: Same as first input
  correct flow6 : Product  Inputs=**  SaturateOnIntegerOverflow=on  RndMeth=Zero  InputSameDT=on  OutDataTypeStr=Inherit: Same as first input
  four : Constant  Value=4  OutDataTypeStr=single  SampleTime=sample_time
      settings: AttributesFormatString=%<Value>\n%<SampleTime>
  svrthrottle1 : Constant  Value=c_svrthrottle1  OutDataTypeStr=single  SampleTime=sample_time
      settings: AttributesFormatString=%<Value>\n%<SampleTime>
  svrthrottle2 : Constant  Value=c_svrthrottle2  OutDataTypeStr=single  SampleTime=sample_time
      settings: AttributesFormatString=%<Value>\n%<SampleTime>
  svrthrottlearg : Constant  Value=c_svrthrottlearg  OutDataTypeStr=single  SampleTime=sample_time
      settings: AttributesFormatString=%<Value>\n%<SampleTime>
  svrthrottleargbeta : Constant  Value=c_svrthrottlebeta  OutDataTypeStr=single  SampleTime=sample_time
      settings: AttributesFormatString=%<Value>\n%<SampleTime>
  tokgps2 : Gain  Gain=1000
  two : Constant  Value=2  OutDataTypeStr=single  SampleTime=sample_time
      settings: AttributesFormatString=%<Value>\n%<SampleTime>
  p_pre_throttle : Outport  OutDataTypeStr=single
  wires:
  Cal_phi/1(phi) -> Saturation3/1
  Pm/1 -> Sum4/2, c_p4d1p4/1, correct flow6/1, correct flow6/2, [Pin]
  Ro_a/1 -> Cal_phi/1(Ro_a)
  Mux/1 -> For_Iterator_Subsystem/1(u)
  TA_deg/1 -> Gain/1
  Gain/1 -> Mux/1
  Gain1/1 -> Mux/2
  Ne_rpm/1 -> Gain1/1
  wegrthr/1 -> tokgps2/1
  tokgps2/1 -> correct flow1/1
  correct flow1/1 -> correct flow2/1, correct flow2/2, Saturation1/1
  four/1 -> correct flow3/1
  c_km1d2k/1 -> correct flow3/3, Saturation7/1
  correct flow3/1 -> Sum1/2
  Sum1/1 -> Saturation/1
  Sqrt/1 -> Sum2/1
  Sum2/1 -> correct flow5/1
  two/1 -> Saturation4/1
  Switch2/1 -> Gain2/1
  Gain2/1 -> p_pre_throttle/1
  correct flow4/1 -> Sum1/1
  Saturation1/1 -> PmbyPa2/2
  Saturation2/1 -> correct flow1/2
  Saturation3/1 -> correct flow1/3
  Saturation7/1 -> correct flow5/2
  Saturation4/1 -> correct flow5/3
  For_Iterator_Subsystem/1(ba) -> Saturation2/1
  Sum4/1 -> [B]
  [B] -> correct flow4/1, correct flow4/2
  [B] -> Sum2/2
  [Pin] -> PmbyPa2/1
  correct flow2/1 -> [Ti]
  [Ti] -> Switch2/3
  [Ti] -> Sum3/1
  correct flow5/1 -> [pp1]
  [pp1] -> Switch2/1
  Sum3/1 -> correct flow3/2
  Saturation/1 -> Sqrt/1
  svrthrottle1/1 -> For_Iterator_Subsystem/2(sv1)
  svrthrottle2/1 -> For_Iterator_Subsystem/3(sv2)
  svrthrottlearg/1 -> For_Iterator_Subsystem/4(arg)
  svrthrottleargbeta/1 -> For_Iterator_Subsystem/5(beta)
  Sum5/1 -> Sum3/2
  correct flow6/1 -> c_km1d2k1/1, Sum5/1
  c_1d2p4/1 -> Relational Operator2/2
  PmbyPa2/1 -> Relational Operator2/1
  Relational Operator2/1 -> Switch2/2
  c_p4d1p4/1 -> Sum4/1
  c_km1d2k1/1 -> Sum5/2

== system KD_cl_harness_tomasso/EGR Throttle/EGR Throttle/Throttle Model2/Air Model_map_use/Back-Flow/Cal phi1 ==
  Pm : Inport
  Ro_m : Inport  Port=2
  Gain2 : Gain  Gain=1/(const.Pcab*const.Pcab/const.Rair/const.Tcab)  SaturateOnIntegerOverflow=on  OutDataTypeStr=Inherit: Same as input  ParamDataTypeStr=Inherit: Same as input
  Math Function : Sqrt  Operator=signedSqrt  AlgorithmType=Newton-Raphson  SaturateOnIntegerOverflow=on
  Product4 : Product  Inputs=**  SaturateOnIntegerOverflow=on  RndMeth=Zero  InputSameDT=on  OutDataTypeStr=Inherit: Same as first input
  phi : Outport
  wires:
  Math Function/1 -> phi/1
  Ro_m/1 -> Product4/2
  Pm/1 -> Product4/1
  Gain2/1 -> Math Function/1
  Product4/1 -> Gain2/1

== system KD_cl_harness_tomasso/EGR Throttle/EGR Throttle/Throttle Model2/Air Model_map_use/Forward-Flow/Cal phi ==
  Pa : Inport
  Ro_a : Inport  Port=2
  Gain2 : Gain  Gain=1/(const.Pcab*const.Pcab/const.Rair/const.Tcab)  SaturateOnIntegerOverflow=on  OutDataTypeStr=Inherit: Same as input  ParamDataTypeStr=Inherit: Same as input
  Math Function : Sqrt  Operator=signedSqrt  AlgorithmType=Newton-Raphson  SaturateOnIntegerOverflow=on
  Product4 : Product  Inputs=**  SaturateOnIntegerOverflow=on  RndMeth=Zero  InputSameDT=on  OutDataTypeStr=Inherit: Same as first input
  phi : Outport
  wires:
  Math Function/1 -> phi/1
  Ro_a/1 -> Product4/2
  Pa/1 -> Product4/1
  Gain2/1 -> Math Function/1
  Product4/1 -> Gain2/1

== system KD_cl_harness_tomasso/EGR Valve/SVR EGR/EGR_model/Air Model_map_use/Back-Flow/Cal phi1 ==
  Pm : Inport
  Ro_m : Inport  Port=2
  Gain2 : Gain  Gain=1/(const.Pcab*const.Pcab/const.Rair/const.Tcab)  SaturateOnIntegerOverflow=on  OutDataTypeStr=Inherit: Same as input  ParamDataTypeStr=Inherit: Same as input
  Math Function : Sqrt  Operator=signedSqrt  AlgorithmType=Newton-Raphson  SaturateOnIntegerOverflow=on
  Product4 : Product  Inputs=**  SaturateOnIntegerOverflow=on  RndMeth=Zero  InputSameDT=on  OutDataTypeStr=Inherit: Same as first input
  phi : Outport
  wires:
  Product4/1 -> Gain2/1
  Gain2/1 -> Math Function/1
  Pm/1 -> Product4/1
  Ro_m/1 -> Product4/2
  Math Function/1 -> phi/1

== system KD_cl_harness_tomasso/EGR Valve/SVR EGR/EGR_model/Air Model_map_use/Forward-Flow/Cal phi ==
  Pa : Inport
  Ro_a : Inport  Port=2
  Gain2 : Gain  Gain=1/(const.Pcab*const.Pcab/const.Rair/const.Tcab)  SaturateOnIntegerOverflow=on  OutDataTypeStr=Inherit: Same as input  ParamDataTypeStr=Inherit: Same as input
  Math Function : Sqrt  Operator=signedSqrt  AlgorithmType=Newton-Raphson  SaturateOnIntegerOverflow=on
  Product4 : Product  Inputs=**  SaturateOnIntegerOverflow=on  RndMeth=Zero  InputSameDT=on  OutDataTypeStr=Inherit: Same as first input
  phi : Outport
  wires:
  Product4/1 -> Gain2/1
  Gain2/1 -> Math Function/1
  Pa/1 -> Product4/1
  Ro_a/1 -> Product4/2
  Math Function/1 -> phi/1

== system KD_cl_harness_tomasso/ctrl_rb_explicit_20131031_v2/expcon/find_region/find_region/leq_check/new_region ==
  rv_in : Inport
  region_in : Inport  Port=2
  Action Port : ActionPort  ActionType=then
  rv_out : Outport
  region_out : Outport  Port=2
  wires:
  rv_in/1 -> rv_out/1
  region_in/1 -> region_out/1

== system KD_cl_harness_tomasso/ctrl_rb_explicit_20131031_v2/expcon/find_region/find_region/leq_check/old_region ==
  rv_in : Inport
  region_in : Inport  Port=2
  Action Port : ActionPort  ActionType=else
  rv_out : Outport
  region_out : Outport  Port=2
  wires:
  rv_in/1 -> rv_out/1
  region_in/1 -> region_out/1
